simulink model "energy"  (R2019a)
settings: Solver=VariableStepAuto  StartTime=0.0  StopTime=200  RelTol=1e-3
libraries: drivingcycle_lib x1
settings Model: Creator=Vaishnav  LastModifiedBy=Vaishnav

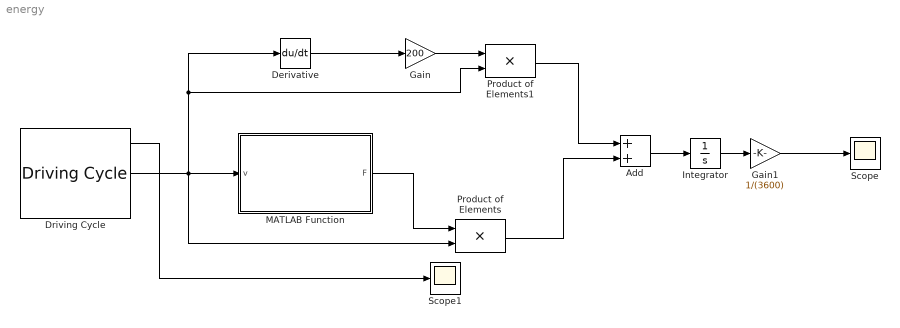
== system energy ==
  Add : Sum
  Derivative : Derivative
  Driving Cycle : drivingcycle_lib/Driving Cycle  CycleName=ECE R15  CycleRepeatsForever=on
      settings: SourceProductName=Driving Cycle Blockset
  Gain : Gain  Gain=200
  Gain1 : Gain  Gain=1/(3600)
  Integrator : Integrator
  MATLAB Function : MATLAB Function  TreatAsAtomicUnit=on
  Product of Elements : Product
  Product of Elements1 : Product
  Scope : Scope
  Scope1 : Scope
  wires:
  MATLAB Function/1(F) -> Product of Elements/1
  Derivative/1 -> Gain/1
  Gain/1 -> Product of Elements1/1
  Product of Elements1/1 -> Add/1
  Product of Elements/1 -> Add/2
  Add/1 -> Integrator/1
  Driving Cycle/2 -> Product of Elements/2, Derivative/1, Product of Elements1/2, MATLAB Function/1(v)
  Driving Cycle/1 -> Scope1/1
  Gain1/1 -> Scope/1
  Integrator/1 -> Gain1/1

== matlab function energy/MATLAB Function ==
  data: v input; F output
function F = fcn(v)

mv = 200;
g = 9.81;
grad = 0.05;
alpha = atan(grad);
Cd = 0.68;
Af = 0.65;
rho = 1.2;
Crr = 0.004;
Fs = mv*g*sin(alpha);
Fr = mv*g*Crr*cos(alpha);
Fa = 0.5*rho*Cd*Af*(v^2);
F = Fs + Fr + Fa;
